simulink model "untitled"  (R2016b)
settings: Solver=VariableStepAuto  StartTime=0.0  StopTime=50.0  RelTol=1e-3
values from neighbouring files (symbols this model uses):
  A = [0 7 2; 0 1 2; 4 2 5]    [t8.m]
  B = [2; 0; 0]    [t8.m]
  C = [2 3 1]    [t8.m]
  D = 0    [t8.m]
  K = place(A,B,[-1; -5; -48])    [t8.m]
settings Model: Creator=mebuffet  LastModifiedBy=mebuffet

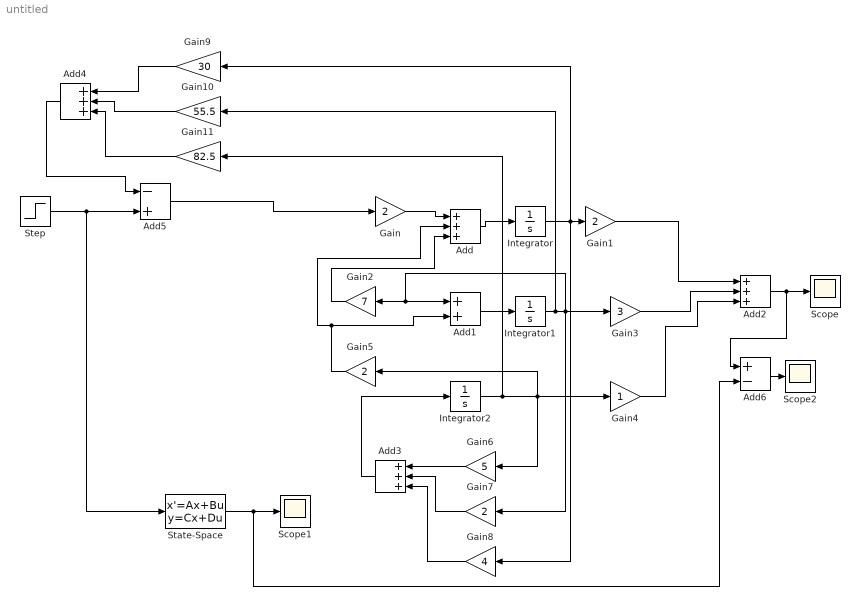
== system untitled ==
  Add{,2..4} (4 alike) : Sum  Inputs=+++
  Add1 : Sum
  Add5 : Sum  Inputs=-+
  Add6 : Sum  Inputs=+-
  Gain{,1,5,7} (4 alike) : Gain  Gain=2
  Gain10 : Gain  Gain=55.5
  Gain11 : Gain  Gain=82.5
  Gain2 : Gain  Gain=7
  Gain3 : Gain  Gain=3
  Gain4 : Gain
  Gain6 : Gain  Gain=5
  Gain8 : Gain  Gain=4
  Gain9 : Gain  Gain=30
  Integrator : Integrator
  Integrator1 : Integrator
  Integrator2 : Integrator
  Scope : Scope
  Scope1 : Scope
  Scope2 : Scope
  State-Space : StateSpace  A=A-B*K  B=B  C=C  D=D  X0=0
  Step : Step  SampleTime=0
  wires:
  Gain/1 -> Add/1
  Add/1 -> Integrator/1
  Gain1/1 -> Add2/1
  Integrator/1 -> Gain9/1, Gain8/1, Gain1/1
  Add2/1 -> Add6/1, Scope/1
  Add1/1 -> Integrator1/1
  Integrator1/1 -> Gain10/1, Gain7/1, Gain3/1, Gain2/1, Add1/1
  Gain3/1 -> Add2/2
  Gain4/1 -> Add2/3
  Integrator2/1 -> Gain11/1, Gain6/1, Gain5/1, Gain4/1
  Gain6/1 -> Add3/1
  Gain7/1 -> Add3/2
  Gain8/1 -> Add3/3
  Add3/1 -> Integrator2/1
  Gain2/1 -> Add/3
  Gain5/1 -> Add1/2, Add/2
  Gain9/1 -> Add4/1
  Gain10/1 -> Add4/2
  Gain11/1 -> Add4/3
  Add4/1 -> Add5/1
  Step/1 -> State-Space/1, Add5/2
  Add5/1 -> Gain/1
  State-Space/1 -> Add6/2, Scope1/1
  Add6/1 -> Scope2/1
